simulink model "SVM_2L_0127210"  (R2023a)
settings: Solver=VariableStepAuto  StartTime=0.0  StopTime=0.1  FixedStep=1e-6  RelTol=1e-3
InitFcn:
  | f=1000;
  | Ts=1/f;
  | Vdc=100;
  | 
  | m=0.9;
libraries: spsSeriesRLCBranchLib x10, spsDCVoltageSourceLib x1, spsPLL3phLib x1, spsThreePhaseVIMeasurementLib x1, spsUniversalBridgeLib x1, spsVoltageMeasurementLib x1, spsabctoAlphaBetaZeroLib x1, spspowerguiLib x1, simulink x1
settings Model: Creator=chen  LastModifiedBy=chen
settings DataIOCC: ReturnWorkspaceOutputs=off
settings DebuggingCC: UnconnectedInputMsg=warning  UnconnectedOutputMsg=warning  UnconnectedLineMsg=warning
settings ModelReferenceCC: EnableRefExpFcnMdlSchedulingChecks=on
settings RTWCC: DLArmComputeVersion=19.05

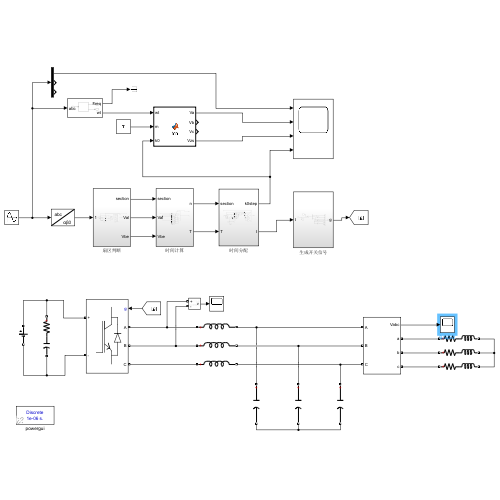
[thumbnail: Simulink's stored preview of the top-level diagram]
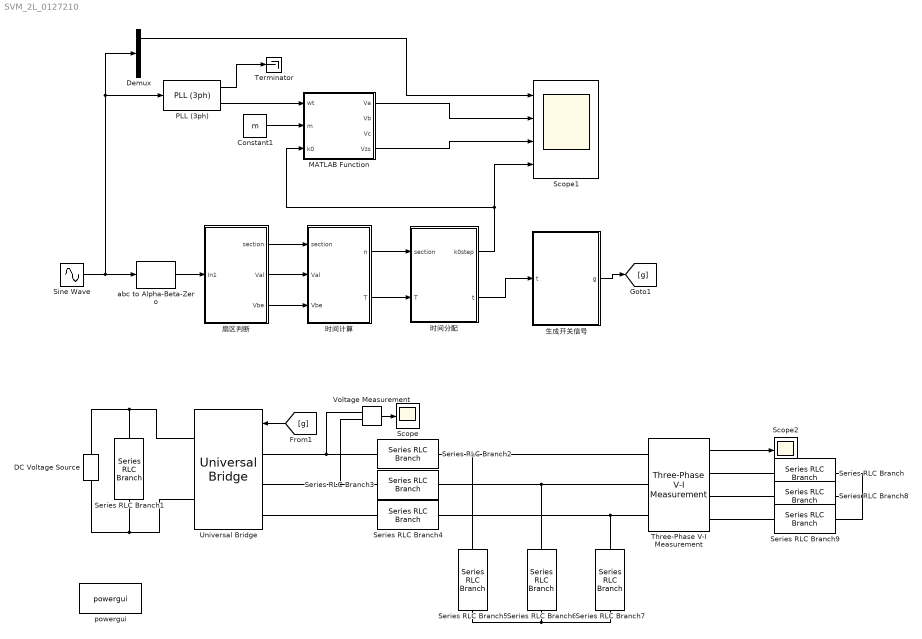
== system SVM_2L_0127210 ==
  Constant1 : Constant  Value=m  SampleTime=0.1
  DC Voltage Source : spsDCVoltageSourceLib/DC Voltage Source  Amplitude=Vdc  Measurements=None
  Demux : Demux  Outputs=3
  MATLAB Function : MATLAB Function  TreatAsAtomicUnit=on
  PLL (3ph) : spsPLL3phLib/PLL (3ph)  Fmin=45  Par_Init=[0, 60]  ParK=[180, 3200, 1]  TcD=1e-4  MaxRateChangeFreq=12  FilterCutOffFreq=25  Ts=0  AGC=on
  Scope : Scope
  Scope1 : Scope  NumInputPorts=4
  Scope2 : Scope
  Series RLC Branch : spsSeriesRLCBranchLib/Series RLC Branch  LConnTagsString=__new0  RConnTagsString=__new0  BranchType=RL  Resistance=10  Inductance=1e-3  SetiL0=off  InitialCurrent=0  Capacitance=1e-6  Setx0=off  InitialVoltage=0  Measurements=None
  Series RLC Branch1 : spsSeriesRLCBranchLib/Series RLC Branch  LConnTagsString=__new0  RConnTagsString=__new0  BranchType=RC  Resistance=1e-6  Inductance=1e-3  SetiL0=off  InitialCurrent=0  Capacitance=1e-6  Setx0=off  InitialVoltage=0  Measurements=None
  Series RLC Branch2 : spsSeriesRLCBranchLib/Series RLC Branch  LConnTagsString=__new0  RConnTagsString=__new0  BranchType=L  Resistance=1  Inductance=6e-3  SetiL0=off  InitialCurrent=0  Capacitance=1e-6  Setx0=off  InitialVoltage=0  Measurements=None
  Series RLC Branch3 : spsSeriesRLCBranchLib/Series RLC Branch  LConnTagsString=__new0  RConnTagsString=__new0  BranchType=L  Resistance=1  Inductance=6e-3  SetiL0=off  InitialCurrent=0  Capacitance=1e-6  Setx0=off  InitialVoltage=0  Measurements=None
  Series RLC Branch4 : spsSeriesRLCBranchLib/Series RLC Branch  LConnTagsString=__new0  RConnTagsString=__new0  BranchType=L  Resistance=1  Inductance=6e-3  SetiL0=off  InitialCurrent=0  Capacitance=1e-6  Setx0=off  InitialVoltage=0  Measurements=None
  Series RLC Branch5 : spsSeriesRLCBranchLib/Series RLC Branch  LConnTagsString=__new0  RConnTagsString=__new0  BranchType=C  Resistance=1  Inductance=1e-3  SetiL0=off  InitialCurrent=0  Capacitance=30e-6  Setx0=off  InitialVoltage=0  Measurements=None
  Series RLC Branch6 : spsSeriesRLCBranchLib/Series RLC Branch  LConnTagsString=__new0  RConnTagsString=__new0  BranchType=C  Resistance=1  Inductance=1e-3  SetiL0=off  InitialCurrent=0  Capacitance=30e-6  Setx0=off  InitialVoltage=0  Measurements=None
  Series RLC Branch7 : spsSeriesRLCBranchLib/Series RLC Branch  LConnTagsString=__new0  RConnTagsString=__new0  BranchType=C  Resistance=1  Inductance=1e-3  SetiL0=off  InitialCurrent=0  Capacitance=30e-6  Setx0=off  InitialVoltage=0  Measurements=None
  Series RLC Branch8 : spsSeriesRLCBranchLib/Series RLC Branch  LConnTagsString=__new0  RConnTagsString=__new0  BranchType=RL  Resistance=10  Inductance=1e-3  SetiL0=off  InitialCurrent=0  Capacitance=1e-6  Setx0=off  InitialVoltage=0  Measurements=None
  Series RLC Branch9 : spsSeriesRLCBranchLib/Series RLC Branch  LConnTagsString=__new0  RConnTagsString=__new0  BranchType=RL  Resistance=10  Inductance=1e-3  SetiL0=off  InitialCurrent=0  Capacitance=1e-6  Setx0=off  InitialVoltage=0  Measurements=None
  Sine Wave : Sin  Amplitude=m  Frequency=2*pi*50  Phase=[0 -2*pi/3 2*pi/3]  SampleTime=0
  Terminator : Terminator
  Three-Phase V-I Measurement : spsThreePhaseVIMeasurementLib/Three-Phase V-I Measurement  VoltageMeasurement=phase-to-phase  SetLabelV=off  LabelV=Vabc  Vpu=off  VpuLL=off  CurrentMeasurement=no  SetLabelI=off  LabelI=Iabc  Ipu=off  Pbase=100e6  Vbase=500e3  OutputType=Complex  PhasorSimulation=off  PSBequivalent=0
  Universal Bridge : spsUniversalBridgeLib/Universal Bridge  Arms=3  SnubberResistance=1e5  SnubberCapacitance=inf  Device=IGBT / Diodes  Ron=1e-3  Lon=0  ForwardVoltages="[  0  0  ]"  ForwardVoltage=0  GTOparameters=[ 10e-6 , 20e-6 ]  IGBTparameters=[ 1e-6 , 2e-6 ]  Measurements=None  Measurements_2=None  converterType=Rectifier
  Voltage Measurement : spsVoltageMeasurementLib/Voltage Measurement  PhasorSimulation=off  OutputType=Complex  PSBequivalent=0
  abc to Alpha-Beta-Zero : spsabctoAlphaBetaZeroLib/abc to Alpha-Beta-Zero
  powergui : spspowerguiLib/powergui  Priority=1  SimulationMode=Discrete  SampleTime=1e-6  frequency=60  Iterations=50  frequencyindice=0  Pbase=100e6  ErrMax=1e-4  UnitsV=kV  UnitsW=MW  buscounter=0  FunctionMessages=off  echomessages=off  EnableUseOfTLC=off  CurrentSourceSwitches=off  DisableSnubberDevices=off  DisableRonSwitches=off  DisableVfSwitches=off  DisplayEquations=off  AutomaticDiscreteSolvers=off  SolverType=Tustin/Backward Euler (TBE)  Interpol=off  ExternalGateDelay=off  methode=off  Ts=100  x0status=blocks  SPID=on  SwTol=0  HookPort=off  NonlinearTolerance=1e-4  nMaxIteration=100  ContinueOnMaxIteration=off  RestoreLinks=warning  ResistiveCurrentMeasurement=off  Frange=[0:2:500]  Ylog=off  Xlog=on  ShowGrid=off  save=off  variable=ZData  structure=0  ZoomFFT=off  StartTime=0.0  cycles=1  DisplayStyle=1  fundamental=60  FreqAxis=off  MaxFrequency=1000  frequencyindicesteady=1  RmsSteady=1  display=off
  扇区判断 : Subsystem
  时间分配 : Subsystem
  时间计算 : Subsystem
  生成开关信号 : Subsystem
  wires:
  Sine Wave/1 -> Demux/1, PLL (3ph)/1, abc to Alpha-Beta-Zero/1
  Three-Phase V-I Measurement/1 -> Scope2/1
  abc to Alpha-Beta-Zero/1 -> 扇区判断/1(In1)
  扇区判断/2(Val) -> 时间计算/2(Val)
  扇区判断/3(Vbe) -> 时间计算/3(Vbe)
  时间计算/2(T) -> 时间分配/2(T)
  扇区判断/1(section) -> 时间计算/1(section)
  时间计算/1(n) -> 时间分配/1(section)
  [g] -> Universal Bridge/1
  时间分配/2(t) -> 生成开关信号/1(t)
  生成开关信号/1(g) -> [g]
  Voltage Measurement/1 -> Scope/1
  PLL (3ph)/1 -> Terminator/1
  PLL (3ph)/2 -> MATLAB Function/1(wt)
  MATLAB Function/1(Va) -> Scope1/2
  Demux/1 -> Scope1/1
  MATLAB Function/4(Vzs) -> Scope1/3
  Constant1/1 -> MATLAB Function/2(m)
  时间分配/1(k0step) -> Scope1/4, MATLAB Function/3(k0)
  connections:
  Series RLC Branch5/RConn1 -- Series RLC Branch7/RConn1 -- Series RLC Branch6/RConn1
  Series RLC Branch/RConn1 -- Series RLC Branch9/RConn1 -- Series RLC Branch8/RConn1
  DC Voltage Source/RConn1 -- Series RLC Branch1/LConn1 -- Universal Bridge/RConn1
  Universal Bridge/RConn2 -- DC Voltage Source/LConn1 -- Series RLC Branch1/RConn1
  Series RLC Branch4/RConn1 -- Three-Phase V-I Measurement/LConn3 -- Series RLC Branch7/LConn1
  Series RLC Branch5/LConn1 -- Three-Phase V-I Measurement/LConn1 -- Series RLC Branch2/RConn1
  Series RLC Branch6/LConn1 -- Three-Phase V-I Measurement/LConn2 -- Series RLC Branch3/RConn1
  Series RLC Branch2/LConn1 -- Voltage Measurement/LConn1 -- Universal Bridge/LConn1
  Universal Bridge/LConn2 -- Voltage Measurement/LConn2 -- Series RLC Branch3/LConn1
  Universal Bridge/LConn3 -- Series RLC Branch4/LConn1
  Series RLC Branch/LConn1 -- Three-Phase V-I Measurement/RConn1
  Three-Phase V-I Measurement/RConn2 -- Series RLC Branch8/LConn1
  Three-Phase V-I Measurement/RConn3 -- Series RLC Branch9/LConn1

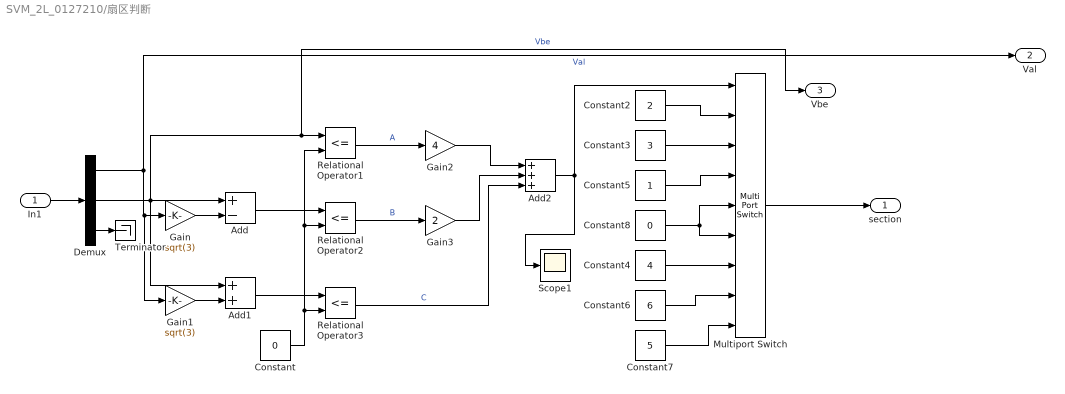
== system SVM_2L_0127210/扇区判断 ==
  In1 : Inport
  Add : Sum  Inputs=+-
  Add1 : Sum
  Add2 : Sum  Inputs=+++
  Constant : Constant  Value=0
  Constant2 : Constant  Value=2
  Constant3 : Constant  Value=3
  Constant4 : Constant  Value=4
  Constant5 : Constant
  Constant6 : Constant  Value=6
  Constant7 : Constant  Value=5
  Constant8 : Constant  Value=0
  Demux : Demux  Outputs=3
  Gain : Gain  Gain=sqrt(3)
  Gain1 : Gain  Gain=sqrt(3)
  Gain2 : Gain  Gain=4
  Gain3 : Gain  Gain=2
  Multiport Switch : MultiPortSwitch  DataPortOrder=Zero-based contiguous  Inputs=8  zeroidx=on  SaturateOnIntegerOverflow=off  InputSameDT=off
  Relational Operator1 : RelationalOperator  Operator=<=  OutDataTypeStr=boolean  RndMeth=Simplest  InputSameDT=off
  Relational Operator2 : RelationalOperator  Operator=<=  OutDataTypeStr=boolean  RndMeth=Simplest  InputSameDT=off
  Relational Operator3 : RelationalOperator  Operator=<=  OutDataTypeStr=boolean  RndMeth=Simplest  InputSameDT=off
  Scope1 : Scope
  Terminator : Terminator
  section : Outport
  Val : Outport  Port=2
  Vbe : Outport  Port=3
  wires:
  Demux/2 -> Add1/1, Add/1, Vbe/1, Relational Operator1/1  "Vbe"
  Constant4/1 -> Multiport Switch/7
  Demux/1 -> Val/1, Gain1/1, Gain/1  "Val"
  Constant8/1 -> Multiport Switch/6, Multiport Switch/5
  Constant7/1 -> Multiport Switch/9
  Add2/1 -> Scope1/1, Multiport Switch/1
  Constant3/1 -> Multiport Switch/3
  Constant5/1 -> Multiport Switch/4
  Constant6/1 -> Multiport Switch/8
  Constant2/1 -> Multiport Switch/2
  Relational Operator1/1 -> Gain2/1  "A"
  Multiport Switch/1 -> section/1
  Relational Operator3/1 -> Add2/3  "C"
  Gain2/1 -> Add2/1
  Gain3/1 -> Add2/2
  Constant/1 -> Relational Operator1/2, Relational Operator2/2, Relational Operator3/2
  Relational Operator2/1 -> Gain3/1  "B"
  Gain/1 -> Add/2
  Gain1/1 -> Add1/2
  Add1/1 -> Relational Operator3/1
  Add/1 -> Relational Operator2/1
  Demux/3 -> Terminator/1
  In1/1 -> Demux/1

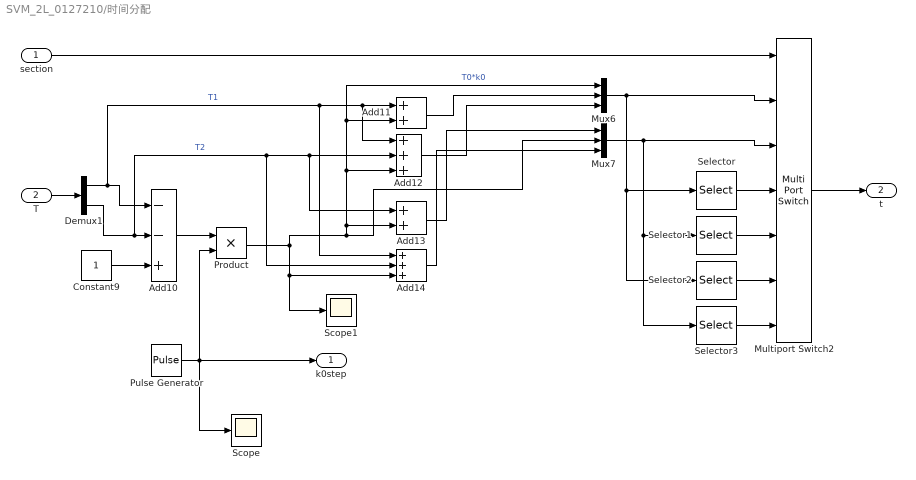
== system SVM_2L_0127210/时间分配 ==
  section : Inport
  T : Inport  Port=2
  Add10 : Sum  Inputs=--+
  Add11 : Sum
  Add12 : Sum  Inputs=+++
  Add13 : Sum
  Add14 : Sum  Inputs=+++
  Constant9 : Constant
  Demux1 : Demux  Outputs=2
  Multiport Switch2 : MultiPortSwitch  Inputs=6  SaturateOnIntegerOverflow=off  InputSameDT=off
  Mux6 : Mux  Inputs=3
  Mux7 : Mux  Inputs=3
  Product : Product
  Pulse Generator : DiscretePulseGenerator  PulseType=Time based  Period=1/150  PulseWidth=50
  Scope : Scope
  Scope1 : Scope
  Selector : Selector  InputPortWidth=3  IndexOptions=Index vector (dialog)  Indices=[3 1 2]  OutputSizes=1
  Selector1 : Selector  InputPortWidth=3  IndexOptions=Index vector (dialog)  Indices=[3 1 2]  OutputSizes=1
  Selector2 : Selector  InputPortWidth=3  IndexOptions=Index vector (dialog)  Indices=[2 3 1]  OutputSizes=1
  Selector3 : Selector  InputPortWidth=3  IndexOptions=Index vector (dialog)  Indices=[2 3 1]  OutputSizes=1
  k0step : Outport
  t : Outport  Port=2
  wires:
  Selector/1 -> Multiport Switch2/4
  Mux6/1 -> Multiport Switch2/2, Selector2/1, Selector/1
  Add11/1 -> Mux6/2
  Product/1 -> Scope1/1, Add14/3, Mux7/2, Add12/3, Add11/2, Mux6/1, Add13/2  "T0*k0"
  Selector2/1 -> Multiport Switch2/6
  Demux1/2 -> Add14/2, Add13/1, Add12/2, Add10/2  "T2"
  Constant9/1 -> Add10/3
  Add14/1 -> Mux7/3
  Mux7/1 -> Selector3/1, Selector1/1, Multiport Switch2/3
  Selector3/1 -> Multiport Switch2/7
  Add13/1 -> Mux7/1
  Selector1/1 -> Multiport Switch2/5
  section/1 -> Multiport Switch2/1
  Demux1/1 -> Add14/1, Add12/1, Add11/1, Add10/1  "T1"
  T/1 -> Demux1/1
  Add10/1 -> Product/1
  Add12/1 -> Mux6/3
  Multiport Switch2/1 -> t/1
  Pulse Generator/1 -> Scope/1, k0step/1, Product/2

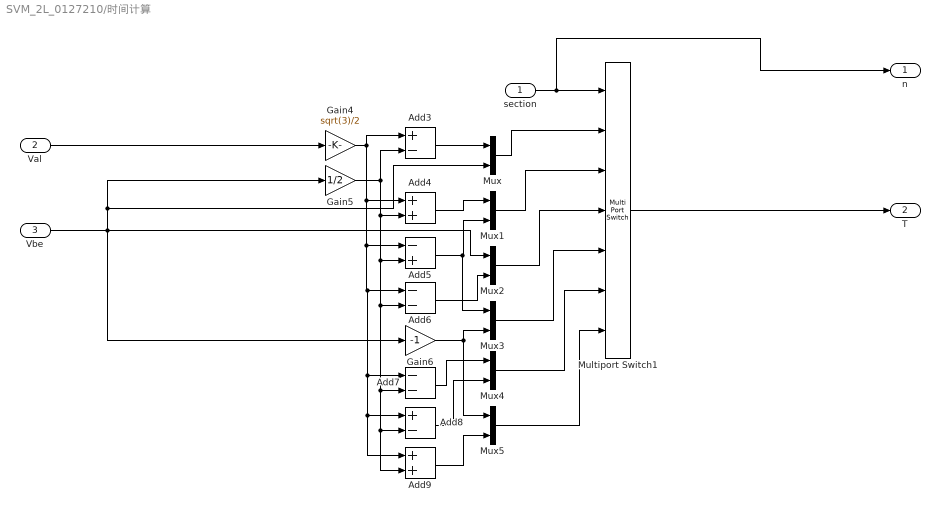
== system SVM_2L_0127210/时间计算 ==
  section : Inport
  Val : Inport  Port=2
  Vbe : Inport  Port=3
  Add3 : Sum  Inputs=+-
  Add4 : Sum
  Add5 : Sum  Inputs=-+
  Add6 : Sum  Inputs=--
  Add7 : Sum  Inputs=--
  Add8 : Sum  Inputs=+-
  Add9 : Sum
  Gain4 : Gain  Gain=sqrt(3)/2
  Gain5 : Gain  Gain=1/2
  Gain6 : Gain  Gain=-1
  Multiport Switch1 : MultiPortSwitch  Inputs=6  SaturateOnIntegerOverflow=off  InputSameDT=off
  Mux{,1..5} (6 alike) : Mux  Inputs=2
  n : Outport
  T : Outport  Port=2
  wires:
  Add8/1 -> Mux4/2
  Gain4/1 -> Add3/1, Add9/1, Add8/1, Add7/1, Add6/1, Add5/1, Add4/1
  Mux2/1 -> Multiport Switch1/4
  Add7/1 -> Mux4/1
  Add9/1 -> Mux5/2
  Mux/1 -> Multiport Switch1/2
  Add3/1 -> Mux/1
  Mux4/1 -> Multiport Switch1/6
  Gain5/1 -> Add5/2, Add6/2, Add8/2, Add9/2, Add7/2, Add4/2, Add3/2
  Add5/1 -> Mux3/1, Mux1/2
  Add4/1 -> Mux1/1
  Mux1/1 -> Multiport Switch1/3
  Mux5/1 -> Multiport Switch1/7
  Val/1 -> Gain4/1
  Vbe/1 -> Gain6/1, Gain5/1, Mux/2, Mux2/1
  Add6/1 -> Mux2/2
  Mux3/1 -> Multiport Switch1/5
  Gain6/1 -> Mux5/1, Mux3/2
  section/1 -> n/1, Multiport Switch1/1
  Multiport Switch1/1 -> T/1

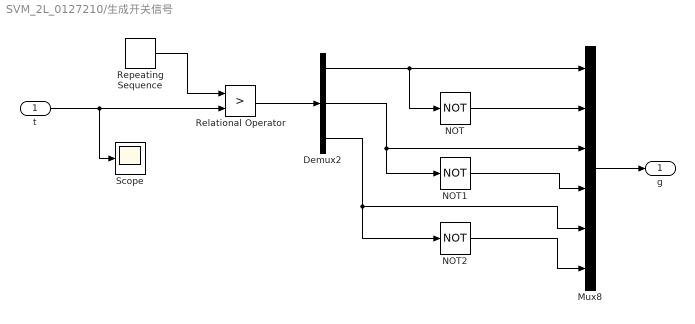
== system SVM_2L_0127210/生成开关信号 ==
  t : Inport
  Demux2 : Demux  Outputs=3
  Mux8 : Mux  Inputs=6
  NOT : Logic  Operator=NOT  IconShape=distinctive  AllPortsSameDT=off  OutDataTypeStr=boolean
  NOT1 : Logic  Operator=NOT  IconShape=distinctive  AllPortsSameDT=off  OutDataTypeStr=boolean
  NOT2 : Logic  Operator=NOT  IconShape=distinctive  AllPortsSameDT=off  OutDataTypeStr=boolean
  Relational Operator : RelationalOperator  Operator=>  OutDataTypeStr=boolean  RndMeth=Simplest  InputSameDT=off
  Repeating Sequence : simulink/Sources/Repeating Sequence  rep_seq_t=[0 Ts/2 Ts]  rep_seq_y=[0 1 0]
  Scope : Scope
  g : Outport
  wires:
  Relational Operator/1 -> Demux2/1
  Demux2/3 -> Mux8/5, NOT2/1
  Demux2/2 -> NOT1/1, Mux8/3
  Demux2/1 -> NOT/1, Mux8/1
  NOT2/1 -> Mux8/6
  NOT/1 -> Mux8/2
  NOT1/1 -> Mux8/4
  Repeating Sequence/1 -> Relational Operator/1
  Mux8/1 -> g/1
  t/1 -> Scope/1, Relational Operator/2

== matlab function SVM_2L_0127210/MATLAB Function ==
  data: wt input; m input; Va output; Vb output; Vc output; Vzs output; k0 input
function [Va,Vb,Vc,Vzs] = fcn(wt, m, k0)
va=m*sin(wt); %m范围0~1
vb=m*sin(wt+pi*2/3); 
vc=m*sin(wt+pi*4/3); 

Vmax=max(va,max(vb,vc));
Vmin=min(va,min(vb,vc));

Vzs=-(Vmax*k0 + Vmin*(1-k0) + (1-2*k0));

Va=va+Vzs;
Vb=vb+Vzs;
Vc=vc+Vzs;
